simulink model "SL7_2_12"  (R2015b)
settings: Solver=VariableStepAuto  StartTime=0.0  StopTime=10.0  RelTol=1e-3
settings Model: Creator=Administrator  LastModifiedBy=Administrator

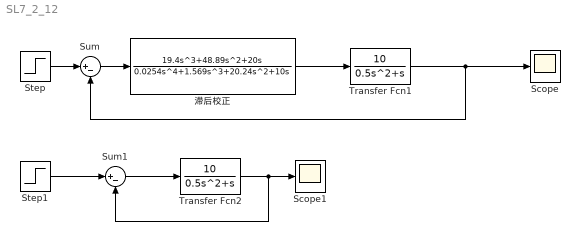
== system SL7_2_12 ==
  Scope : Scope
  Scope1 : Scope
  Step : Step  Time=0  SampleTime=0  VectorParams1D=off
  Step1 : Step  Time=0  SampleTime=0
  Sum : Sum  Inputs=|+-
  Sum1 : Sum  Inputs=|+-
  Transfer Fcn1 : TransferFcn  Numerator=[10]  Denominator=[0.5 1 0]
  Transfer Fcn2 : TransferFcn  Numerator=[10]  Denominator=[0.5 1 0]
  滞后校正 : TransferFcn  Numerator=[19.4 48.89 20 0]  Denominator=[0.0254 1.569 20.24 10 0]
  wires:
  滞后校正/1 -> Transfer Fcn1/1
  Sum/1 -> 滞后校正/1
  Step/1 -> Sum/1
  Transfer Fcn1/1 -> Sum/2, Scope/1
  Transfer Fcn2/1 -> Sum1/2, Scope1/1
  Sum1/1 -> Transfer Fcn2/1
  Step1/1 -> Sum1/1
